simulink model "DynamicModelTransformer_load"  (Simulink 7.8)
settings: Solver=ode45  StartTime=0.0  StopTime=2  MaxStep=0.2e-3  RelTol=1e-6
InitFcn:
  | Omega = 2*pi*50;
  | 
  | Nratio   = 10;
  | 
  | R1       = 0.72;
  | L1lkg   = 0.92/Omega;
  | L1m     = 4370/Omega;
  | L11      = L1m+L1lkg;
  | 
  | R2       = 0.007;
  | L2lkg   = 0.009/Omega;
  | L2m     = 43.7/Omega;
  | L22      = L2m+L2lkg;
  | 
  | M         = L1m/Nratio;
  | 
  | RL       = 0.8962;
  | LL       = 0.6721/Omega;
settings Model: Creator=klu  LastModifiedBy=Fitim k
settings OptimizationCC: InitFltsAndDblsToZero=on
settings DebuggingCC: FcnCallInpInsideContextMsg=Use local settings  StrictBusMsg=Warning

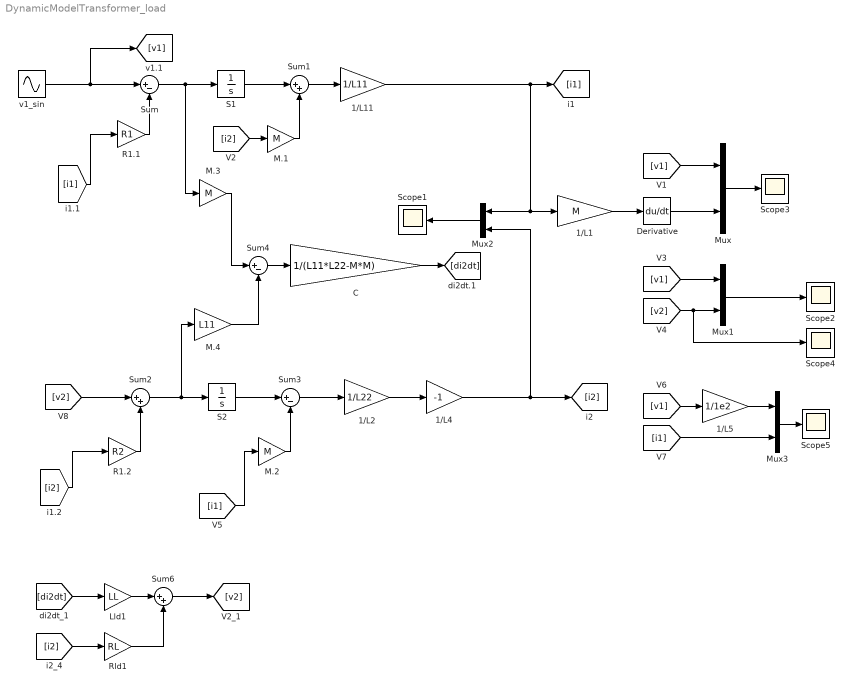
== system DynamicModelTransformer_load ==
  1/L1 : Gain  Gain=M
  1/L11 : Gain  Gain=1/L11
  1/L2 : Gain  Gain=1/L22
  1/L4 : Gain  Gain=-1
  1/L5 : Gain  Gain=1/1e2
  C : Gain  Gain=1/(L11*L22-M*M)
  Derivative : Derivative
  Lld1 : Gain  Gain=LL
  M.1 : Gain  Gain=M
  M.2 : Gain  Gain=M
  M.3 : Gain  Gain=M
  M.4 : Gain  Gain=L11
  Mux{,1..3} (4 alike) : Mux  Inputs=2
  R1.1 : Gain  Gain=R1
  R1.2 : Gain  Gain=R2
  Rld1 : Gain  Gain=RL
  S1 : Integrator
  S2 : Integrator
  Scope{1..5} (5 alike) : Scope
      Scope1 settings: TimeRange=0.05086362794936428  YMin=-0.1  YMax=1.2
      Scope2 settings: TimeRange=0.05179845422116514  YMin=-2957.943925233645  YMax=2705.607476635514
      Scope3 settings: SaveName=ScopeData2
      Scope4 settings: YMin=-100  YMax=100  SaveName=ScopeData3
      Scope5 settings: TimeRange=0.04770744137131677  YMin=-25  YMax=24.89224137931034  SaveName=ScopeData4
  Sum : Sum  Inputs=|+-
  Sum1 : Sum  Inputs=|++
  Sum2 : Sum  Inputs=|++
  Sum3 : Sum  Inputs=|+-
  Sum4 : Sum  Inputs=|+-
  Sum6 : Sum  Inputs=|++
  v1_sin : Sin  Amplitude=2400  Frequency=2*pi*50  Phase=pi/2*0  SampleTime=0
  wires:
  v1_sin/1 -> Sum/1, [v1]
  Sum/1 -> S1/1, M.3/1
  S1/1 -> Sum1/1
  Sum1/1 -> 1/L11/1
  1/L11/1 -> [i1], 1/L1/1, Mux2/1
  R1.1/1 -> Sum/2
  [i1] -> R1.1/1
  M.1/1 -> Sum1/2
  Mux/1 -> Scope3/1
  1/L1/1 -> Derivative/1
  Derivative/1 -> Mux/2
  [v1] -> Mux/1
  Sum2/1 -> S2/1, M.4/1
  S2/1 -> Sum3/1
  Sum3/1 -> 1/L2/1
  R1.2/1 -> Sum2/2
  [i2] -> R1.2/1
  M.2/1 -> Sum3/2
  1/L2/1 -> 1/L4/1
  [i2] -> M.1/1
  Mux1/1 -> Scope2/1
  [v1] -> Mux1/1
  [v2] -> Mux1/2, Scope4/1
  Mux2/1 -> Scope1/1
  1/L4/1 -> [i2], Mux2/2
  [v1] -> 1/L5/1
  1/L5/1 -> Mux3/1
  [i1] -> Mux3/2
  Mux3/1 -> Scope5/1
  M.3/1 -> Sum4/1
  Sum4/1 -> C/1
  C/1 -> [di2dt]
  [i2] -> Rld1/1
  [di2dt] -> Lld1/1
  Lld1/1 -> Sum6/1
  Rld1/1 -> Sum6/2
  Sum6/1 -> [v2]
  [v2] -> Sum2/1
  [i1] -> M.2/1
  M.4/1 -> Sum4/2
